simulink model "vectorscope_tut1"  (Simulink 5.0)
settings: Solver=FixedStepDiscrete  StartTime=0.0  StopTime=inf  RelTol=1e-3
undefined symbols (not defined in the file or in its folder): get
libraries: dspsrcs4 x2, dspspect3 x1, dspsnks4 x1
settings Model: Creator=ckamachi  LastModifiedBy=ckamachi  ExtModeTrigMode=oneshot  ExtModeArmWhenConnect=off  LimitDataPoints=off  BlockReductionOpt=off  BooleanDataType=off

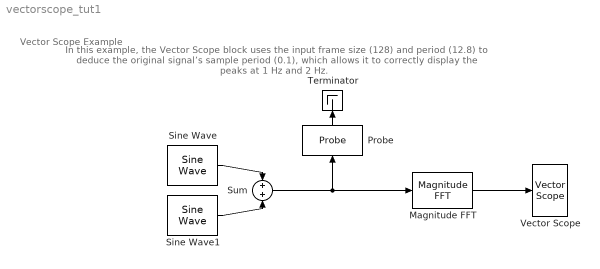
== system vectorscope_tut1 ==
  note: Vector Scope Example
  note: In this example, the Vector Scope block uses the input frame size (128) and
      | period (12.8) to deduce the original signal’s sample period (0.1), which allows
      | it to correctly display the peaks at 1 Hz and 2 Hz.
  Magnitude FFT : dspspect3/Magnitude FFT  mag_or_magsq=Magnitude squared  fftLenInherit=on  fftsize=256
  Probe : Probe  Orientation=up  ProbeWidth=off  ProbeComplexSignal=off
  Sine Wave : dspsrcs4/Sine Wave  Amplitude=1  Frequency=1  Phase=0  SampleMode=Discrete  OutComplex=Real  CompMethod=Trigonometric fcn  TableSize=Speed  SampleTime=0.1  SamplesPerFrame=128  dataType=double  wordLen=16  udDataType=sfix(16)  fracBitsMode=Best precision  numFracBits=14  ResetState=Restart at time zero
  Sine Wave1 : dspsrcs4/Sine Wave  Amplitude=1  Frequency=2  Phase=0  SampleMode=Discrete  OutComplex=Real  CompMethod=Trigonometric fcn  TableSize=Speed  SampleTime=0.1  SamplesPerFrame=128  dataType=double  wordLen=16  udDataType=sfix(16)  fracBitsMode=Best precision  numFracBits=14  ResetState=Restart at time zero
  Sum : Sum  Inputs=+|+  SaturateOnIntegerOverflow=on  InputSameDT=on
  Terminator : Terminator
      settings: Orientation=up
  Vector Scope : dspsnks4/Vector Scope  ScopeProperties=off  Domain=Frequency  HorizSpan=1  DisplayProperties=off  AxisGrid=on  Memory=off  FrameNumber=on  AxisLegend=off  AxisZoom=off  OpenScopeAtSimStart=on  OpenScopeImmediately=off  FigPos=get(0,'defaultfigureposition')  AxisProperties=on  XUnits=Hertz  XRange=[0...Fs/2]  InheritXIncr=on  XIncr=-1  XLabel=Samples  YUnits=dB  YLabel=Amplitude  LineProperties=off
      settings: YMin=-10  YMax=40
  wires:
  Sine Wave/1 -> Sum/1
  Sum/1 -> Probe/1, Magnitude FFT/1
  Magnitude FFT/1 -> Vector Scope/1
  Sine Wave1/1 -> Sum/2
  Probe/1 -> Terminator/1
